simulink model "MSV_ablf"  (R2021a)
settings: Solver=ode4  StartTime=0.0  StopTime=10  FixedStep=0.001  MaxStep=0.01  RelTol=1e-3
model workspace (MAT data in the model file):
  EnableF = 1
  F_xyh = [10; 10; 1]
  GainKnownUncty = 1
  InputSat = [8591; 330.8; 839]
  InputSatOff = 1000
  Mmtx = [1  0  0; 0  1  0; 0  0  1]
  Temp = 0
  Test1 = Simulink.Parameter
  Test1.Value = 0
  Test1.DataType = 'auto'
  Test1.Dimensions = [1 1]
  boat_heading = 0
  boat_vel_x = 0
  boat_vel_y = 0
  earth_head = 2
  earth_x = 0
  earth_y = 2
  input_heading = 1
  input_x = 1
  input_y = 1
values from neighbouring files (symbols this model uses):
  Fval = [0 0 0]    [max_dist.m]    (also in test_ablf.m = [ ix iy iz ]; test_bs.m = [ ix iy iz ]; test_fxt.m = [ ix iy iz ]; test_max.m)
  LimStop = 0    [main.m]    (also in max_dist.m = 1)
libraries: dspmtrx3 x18, aerolibutil x4, simulink x1
(part 1 of 2)
settings Model: PacingRate=0.500000  ParameterArgumentNames=earth_head,earth_x,earth_y  OrderedModelArguments=off  Creator=14244039  LastModifiedBy=14244039
settings DebuggingCC: ReadBeforeWriteMsg=DisableAll
settings RTWCC: GenCodeOnly=on  BuildConfiguration=Faster Runs

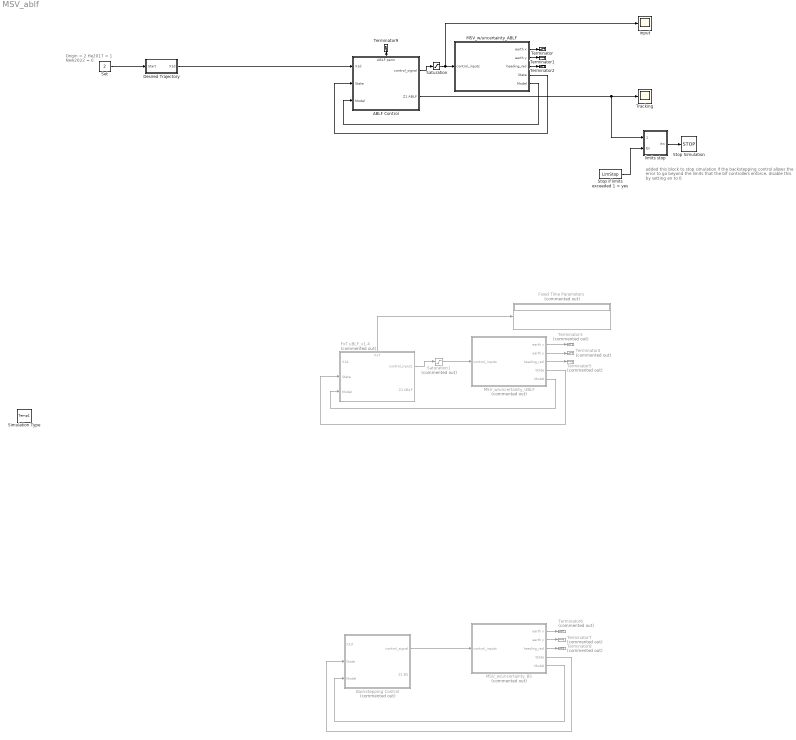
== system MSV_ablf ==
  note: Origin = 2
      | He2017 = 1
      | New2022 = 0
  note: added this block to stop simulation if the backstepping control allows
      | the error to go beyond the limits that the blf controllers enforce.
      | disable this by setting en to 0
  ABLF Control : Subsystem
      settings: PortSchema="{\"entries\":[{\"content\":{\"sides\":[{\"content\":{\"connectorIds\":[\"In1\",\"In2\",\"In3\"]},\"type\":\"ConnectorPlacement.EquallySpacedRectSide\",\"uuid\":\"f8e83fd1-45ec-473c-b127-dda3e39bc690\"},{\"content\":{\"connectorIds\":[\"Out1\",\"Out2\"],\"side\":\"RIGHT\"},\"type\":\"ConnectorPlacement.EquallySpacedRectSide\",\"uuid\":\"3907a693-0eb5-4391-af9e-fb1e42d629e6\"},{\"content\":{\"connectorIds\":[\"Out3\"],\"side\":\"TOP\"},\"type\":\"ConnectorPlacement.EquallySpacedRectSide\",\"uuid\":\"67f51e78-fb2e-4534-9eac-637fb7bc723a\"}]},\"type\":\"ConnectorPlacement.EquallySpacedConnector\",\"uuid\":\"eb746a93-d2ce-4178-8726-02b0a13fef5e\"}],\"packageUris\":[\"http://schema.mathworks.com/mf0/Connector/R2020b\"],\"version\":\"1.0\"}"
  Backstepping Control : Subsystem  Commented=on
  Desired Trajectory : Subsystem
  Fixed Time Parameters : Display  Commented=on
  FxT uBLF_v1.4 : Subsystem  Commented=on
      settings: PortSchema="{\"entries\":[{\"content\":{\"sides\":[{\"content\":{\"connectorIds\":[\"In1\",\"In2\",\"In3\"]},\"type\":\"ConnectorPlacement.EquallySpacedRectSide\",\"uuid\":\"f8e83fd1-45ec-473c-b127-dda3e39bc690\"},{\"content\":{\"connectorIds\":[\"Out1\",\"Out2\"],\"side\":\"RIGHT\"},\"type\":\"ConnectorPlacement.EquallySpacedRectSide\",\"uuid\":\"3907a693-0eb5-4391-af9e-fb1e42d629e6\"},{\"content\":{\"connectorIds\":[\"Out3\"],\"side\":\"TOP\"},\"type\":\"ConnectorPlacement.EquallySpacedRectSide\",\"uuid\":\"67f51e78-fb2e-4534-9eac-637fb7bc723a\"}]},\"type\":\"ConnectorPlacement.EquallySpacedConnector\",\"uuid\":\"eb746a93-d2ce-4178-8726-02b0a13fef5e\"}],\"packageUris\":[\"http://schema.mathworks.com/mf0/Connector/R2020b\"],\"version\":\"1.0\"}"
  MSV_w/uncertainty_ABLF : Subsystem
  MSV_w/uncertainty_BS : Subsystem  Commented=on
  MSV_w/uncertainty_UBLF : Subsystem  Commented=on
  Saturation : Saturate  UpperLimit=InputSat*InputSatOff  LowerLimit=-1*(InputSat)*InputSatOff
  Saturation1 : Saturate  Commented=on  UpperLimit=InputSat*InputSatOff  LowerLimit=-1*(InputSat)*InputSatOff
  Set : Constant  Value=2
  Simulation Type : DataStoreMemory  DataStoreName=Temp1  ReadBeforeWriteMsg=warning  WriteAfterWriteMsg=warning  WriteAfterReadMsg=warning  ShowAdditionalParam=off
  Stop Simulation : Stop
  Stop if limits exceeded 1 = yes : Constant  Value=LimStop
  Terminator{,1..2,9} (4 alike) : Terminator
  Terminator{3..8} (6 alike) : Terminator  Commented=on
  Tracking : Scope
  input : Scope
  limits stop : Subsystem
  wires:
  MSV_w/uncertainty_UBLF/4(State) -> FxT uBLF_v1.4/2(State)
  MSV_w/uncertainty_UBLF/5(Model) -> FxT uBLF_v1.4/3(Model)
  MSV_w/uncertainty_ABLF/4(State) -> ABLF Control/2(State)
  MSV_w/uncertainty_ABLF/5(Model) -> ABLF Control/3(Model)
  Set/1 -> Desired Trajectory/1(Start)
  FxT uBLF_v1.4/1(control_inputs) -> Saturation1/1
  ABLF Control/1(control_signal) -> Saturation/1
  Saturation1/1 -> MSV_w/uncertainty_UBLF/1(control_inputs)
  FxT uBLF_v1.4/3(FxT) -> Fixed Time Parameters/1
  Desired Trajectory/1(X1d) -> ABLF Control/1(X1d)
  Backstepping Control/1(control_signal) -> MSV_w/uncertainty_BS/1(control_inputs)
  MSV_w/uncertainty_BS/5(Model) -> Backstepping Control/3(Model)
  MSV_w/uncertainty_BS/4(State) -> Backstepping Control/2(State)
  MSV_w/uncertainty_ABLF/1(earth x) -> Terminator/1
  MSV_w/uncertainty_ABLF/2(earth y) -> Terminator1/1
  MSV_w/uncertainty_ABLF/3(heading_rad) -> Terminator2/1
  MSV_w/uncertainty_UBLF/1(earth x) -> Terminator3/1
  MSV_w/uncertainty_UBLF/2(earth y) -> Terminator4/1
  MSV_w/uncertainty_UBLF/3(heading_rad) -> Terminator5/1
  MSV_w/uncertainty_BS/1(earth x) -> Terminator6/1
  MSV_w/uncertainty_BS/2(earth y) -> Terminator7/1
  MSV_w/uncertainty_BS/3(heading_rad) -> Terminator8/1
  Saturation/1 -> input/1, MSV_w/uncertainty_ABLF/1(control_inputs)
  ABLF Control/3(ABLF parm) -> Terminator9/1
  limits stop/1(rtn) -> Stop Simulation/1
  ABLF Control/2(Z1 ABLF) -> limits stop/1(Z1 BS), Tracking/1
  Stop if limits exceeded 1 = yes/1 -> limits stop/2(En)

== system MSV_ablf/ABLF Control ==
  X1d : Inport
  State : Inport  Port=2
  Model : Inport  Port=3
  Constant : Constant  Value=0
  MATLAB Function : MATLAB Function  TreatAsAtomicUnit=on
  Selector : Selector  InputPortWidth=3  IndexOptions=Index vector (dialog)  Indices=1  OutputSizes=1
  Selector1 : Selector  InputPortWidth=3  IndexOptions=Index vector (dialog)  Indices=2  OutputSizes=1
  Selector2 : Selector  InputPortWidth=3  IndexOptions=Index vector (dialog)  Indices=3  OutputSizes=1
  State Feedback & Known Functions : Subsystem
  Terminator{,1..3} (4 alike) : Terminator
  u_ablf : Scope  NumInputPorts=3
  control_signal : Outport
  Z1 ABLF : Outport  Port=2
  ABLF parm : Outport  Port=3
  wires:
  State/1 -> State Feedback & Known Functions/2(State)
  State Feedback & Known Functions/1(C+D+G) -> MATLAB Function/1(CDG)
  State Feedback & Known Functions/2(M) -> MATLAB Function/2(M)
  State Feedback & Known Functions/5(X2) -> MATLAB Function/5(X2)
  State Feedback & Known Functions/4(X1) -> MATLAB Function/4(X1)
  State Feedback & Known Functions/3(J) -> MATLAB Function/3(J)
  Model/1 -> State Feedback & Known Functions/1(Model)
  X1d/1 -> MATLAB Function/6(X1d)  "xd"
  MATLAB Function/6(test2) -> Z1 ABLF/1
  MATLAB Function/7(pABLF) -> ABLF parm/1
  Selector/1 -> u_ablf/1  "uLong"
  MATLAB Function/1(u) -> control_signal/1, Selector/1, Selector1/1, Selector2/1
  Selector1/1 -> u_ablf/2  "uLateral"
  Selector2/1 -> u_ablf/3  "uRotate"
  Constant/1 -> MATLAB Function/8(unused1), MATLAB Function/7(unused)
  MATLAB Function/2(x_Err) -> Terminator/1
  MATLAB Function/3(y_Err) -> Terminator1/1
  MATLAB Function/4(h_Err) -> Terminator2/1
  MATLAB Function/5(test1) -> Terminator3/1

== system MSV_ablf/Backstepping Control ==
  X1d : Inport
  State : Inport  Port=2
  Model : Inport  Port=3
  Constant : Constant
  MATLAB Function : MATLAB Function  TreatAsAtomicUnit=on
  Selector : Selector  InputPortWidth=3  IndexOptions=Index vector (dialog)  Indices=1  OutputSizes=1
  Selector1 : Selector  InputPortWidth=3  IndexOptions=Index vector (dialog)  Indices=2  OutputSizes=1
  Selector2 : Selector  InputPortWidth=3  IndexOptions=Index vector (dialog)  Indices=3  OutputSizes=1
  State Feedback & Known Functions : Subsystem
  Terminator{,1..3} (4 alike) : Terminator
  u_bs : Scope  NumInputPorts=3
  control_signal : Outport
  Z1 BS : Outport  Port=2
  wires:
  State/1 -> State Feedback & Known Functions/2(State)
  State Feedback & Known Functions/1(C+D+G) -> MATLAB Function/1(CDG)
  State Feedback & Known Functions/2(M) -> MATLAB Function/2(M)
  State Feedback & Known Functions/5(X2) -> MATLAB Function/5(X2)
  State Feedback & Known Functions/4(X1) -> MATLAB Function/4(X1)
  State Feedback & Known Functions/3(J) -> MATLAB Function/3(J)
  Model/1 -> State Feedback & Known Functions/1(Model)
  X1d/1 -> MATLAB Function/6(X1d)  "xd"
  MATLAB Function/6(test2) -> Z1 BS/1
  Selector/1 -> u_bs/1  "uLong"
  MATLAB Function/1(u) -> Selector/1, Selector1/1, Selector2/1, control_signal/1
  Selector1/1 -> u_bs/2  "uLateral"
  Selector2/1 -> u_bs/3  "uRotate"
  Constant/1 -> MATLAB Function/8(unused1), MATLAB Function/7(unused)
  MATLAB Function/2(x_Err) -> Terminator/1
  MATLAB Function/3(y_Err) -> Terminator1/1
  MATLAB Function/4(h_Err) -> Terminator2/1
  MATLAB Function/5(test1) -> Terminator3/1

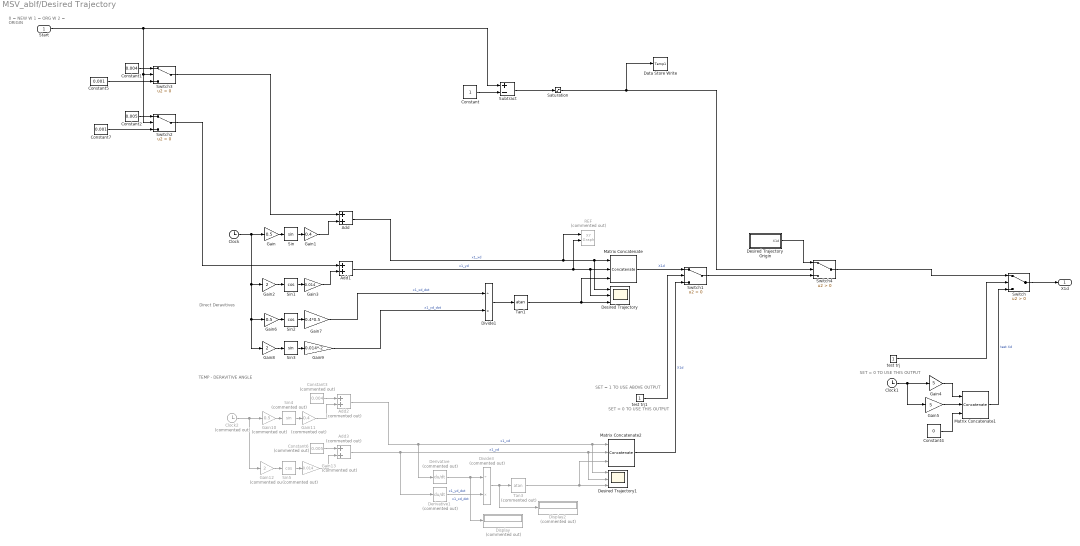
== system MSV_ablf/Desired Trajectory ==
  note: 0 = NEW W
      | 1 = ORG W
      | 2 = ORIGIN
  note: Direct Deravitives
  note: SET = 0 TO USE THIS OUTPUT
  note: TEMP - DERAVITIVE ANGLE
  note: SET = 1 TO USE ABOVE OUTPUT
  note: SET = 0 TO USE THIS OUTPUT
  Start : Inport
  Add : Sum
  Add1 : Sum
  Add2 : Sum  Commented=on
  Add3 : Sum  Commented=on
  Clock : Clock
  Clock1 : Clock
  Clock2 : Clock  Commented=on
  Constant : Constant
  Constant1 : Constant  Value=0.004
  Constant2 : Constant  Value=0.005
  Constant3 : Constant  Commented=on  Value=0.004
  Constant4 : Constant  Value=0
  Constant5 : Constant  Value=0.001
  Constant6 : Constant  Commented=on  Value=0.005
  Constant7 : Constant  Value=0.001
  Data Store Write : DataStoreWrite  DataStoreName=Temp1  IndexOptions=Index vector (dialog)  Indices=1  OutputSizes=1
  Derivative : Derivative  Commented=on
  Derivative1 : Derivative  Commented=on
  Desired Trajectory : Scope  NumInputPorts=3
  Desired Trajectory Origin : Subsystem
  Desired Trajectory1 : Scope  NumInputPorts=3
  Display : Display  Commented=on
  Display2 : Display  Commented=on
  Divide1 : Product  Inputs=/*
  Divide3 : Product  Commented=on  Inputs=/*
  Gain : Gain  Gain=0.5
  Gain1 : Gain  Gain=0.4
  Gain10 : Gain  Commented=on  Gain=0.5
  Gain11 : Gain  Commented=on  Gain=0.4
  Gain12 : Gain  Commented=on  Gain=2
  Gain13 : Gain  Commented=on  Gain=0.014
  Gain2 : Gain  Gain=2
  Gain3 : Gain  Gain=0.014
  Gain4 : Gain  Gain=5
  Gain5 : Gain  Gain=5
  Gain6 : Gain  Gain=0.5
  Gain7 : Gain  Gain=0.4*0.5
  Gain8 : Gain  Gain=2
  Gain9 : Gain  Gain=0.014*-2
  Matrix Concatenate : Concatenate  NumInputs=3  Mode=Multidimensional array
  Matrix Concatenate1 : Concatenate  NumInputs=3  Mode=Multidimensional array
  Matrix Concatenate2 : Concatenate  NumInputs=3  Mode=Multidimensional array
  REF : simulink/Sinks/XY Graph  Commented=on  xmin=-0.65  xmax=0.65  ymin=-0.012  ymax=0.022  st=-1
  Saturation : Saturate  UpperLimit=1
  Sin : Trigonometry
  Sin1 : Trigonometry  Operator=cos
  Sin2 : Trigonometry  Operator=cos
  Sin3 : Trigonometry
  Sin4 : Trigonometry  Commented=on
  Sin5 : Trigonometry  Commented=on  Operator=cos
  Subtract : Sum  Inputs=+-
  Switch{,1..4} (5 alike) : Switch  Criteria=u2 > Threshold
  Tan1 : Trigonometry  Operator=atan  ApproximationMethod=CORDIC  OutputSignalType=real
  Tan3 : Trigonometry  Commented=on  Operator=atan  ApproximationMethod=CORDIC  OutputSignalType=real
  test trj : Constant
  test trj1 : Constant
  X1d : Outport
  wires:
  Clock/1 -> Gain/1, Gain8/1, Gain6/1, Gain2/1
  Switch3/1 -> Add/1
  Sin/1 -> Gain1/1
  Gain/1 -> Sin/1
  Add1/1 -> Matrix Concatenate/2, Desired Trajectory/2, REF/2  "x1_yd"
  Gain1/1 -> Add/2
  Switch2/1 -> Add1/1
  Gain2/1 -> Sin1/1
  Add/1 -> REF/1, Desired Trajectory/1, Matrix Concatenate/1  "x1_xd"
  Gain3/1 -> Add1/2
  Sin1/1 -> Gain3/1
  Matrix Concatenate/1 -> Switch1/1  "X1d"
  Gain9/1 -> Divide1/2  "x1_yd_dot"
  Tan1/1 -> Matrix Concatenate/3, Desired Trajectory/3
  Switch/1 -> X1d/1
  test trj/1 -> Switch/2
  Matrix Concatenate1/1 -> Switch/3  "test Xd"
  Gain5/1 -> Matrix Concatenate1/2
  Gain4/1 -> Matrix Concatenate1/1
  Clock1/1 -> Gain5/1, Gain4/1
  Constant4/1 -> Matrix Concatenate1/3
  Gain7/1 -> Divide1/1  "x1_xd_dot"
  Divide1/1 -> Tan1/1
  Gain6/1 -> Sin2/1
  Sin2/1 -> Gain7/1
  Sin3/1 -> Gain9/1
  Gain8/1 -> Sin3/1
  Divide3/1 -> Display2/1, Tan3/1
  Derivative/1 -> Display/1, Divide3/1  "x1_xd_dot"
  Tan3/1 -> Desired Trajectory1/3, Matrix Concatenate2/3
  Derivative1/1 -> Divide3/2  "x1_yd_dot"
  Sin5/1 -> Gain13/1
  Gain13/1 -> Add3/2
  Add2/1 -> Derivative/1, Matrix Concatenate2/1, Desired Trajectory1/1  "x1_xd"
  Gain12/1 -> Sin5/1
  Constant6/1 -> Add3/1
  Gain11/1 -> Add2/2
  Add3/1 -> Derivative1/1, Matrix Concatenate2/2, Desired Trajectory1/2  "x1_yd"
  Gain10/1 -> Sin4/1
  Sin4/1 -> Gain11/1
  Constant3/1 -> Add2/1
  Clock2/1 -> Gain12/1, Gain10/1
  Switch4/1 -> Switch/1
  Matrix Concatenate2/1 -> Switch1/3  "X1d"
  test trj1/1 -> Switch1/2
  Constant2/1 -> Switch2/1
  Constant1/1 -> Switch3/1
  Constant5/1 -> Switch3/3
  Constant7/1 -> Switch2/3
  Switch1/1 -> Switch4/3
  Desired Trajectory Origin/1(X1d) -> Switch4/1
  Subtract/1 -> Saturation/1
  Constant/1 -> Subtract/2
  Start/1 -> Switch2/2, Switch3/2, Subtract/1
  Saturation/1 -> Data Store Write/1, Switch4/2

== system MSV_ablf/FxT uBLF_v1.4 ==
  X1d : Inport
  State : Inport  Port=2
  Model : Inport  Port=3
  Constant : Constant  Value=0
  Control Signals : Scope  NumInputPorts=3
  Fixed Time Tmax : Display
  Selector : Selector  InputPortWidth=3  IndexOptions=Index vector (dialog)  Indices=1  OutputSizes=1
  Selector1 : Selector  InputPortWidth=3  IndexOptions=Index vector (dialog)  Indices=2  OutputSizes=1
  Selector2 : Selector  InputPortWidth=3  IndexOptions=Index vector (dialog)  Indices=3  OutputSizes=1
  Selector3 : Selector  InputPortWidth=9  IndexOptions=Index vector (dialog)  Indices=1  OutputSizes=1
  State Feedback & Known Functions : Subsystem
  SymUBLF1 : MATLAB Function  Commented=on  TreatAsAtomicUnit=on
  Terminator : Terminator
  Terminator1 : Terminator
  Terminator2 : Terminator
  UBLF : MATLAB Function  TreatAsAtomicUnit=on
  control_inputs : Outport
  Z1 UBLF : Outport  Port=2
  FxT : Outport  Port=3
  wires:
  X1d/1 -> UBLF/6(Xd)  "X1d"
  Model/1 -> State Feedback & Known Functions/1(Model)
  State/1 -> State Feedback & Known Functions/2(State)
  State Feedback & Known Functions/1(F2) -> UBLF/1(F2)
  State Feedback & Known Functions/2(G2) -> UBLF/2(G2)
  State Feedback & Known Functions/3(G1) -> UBLF/3(G1)
  State Feedback & Known Functions/4(X1) -> UBLF/4(X1)
  State Feedback & Known Functions/5(X2) -> UBLF/5(X2)
  Selector/1 -> Control Signals/1  "uLong"
  Selector1/1 -> Control Signals/2  "uLateral"
  Selector2/1 -> Control Signals/3  "uRotate"
  UBLF/1(u) -> control_inputs/1, Selector1/1, Selector2/1, Selector/1
  UBLF/5(test1) -> Z1 UBLF/1
  UBLF/6(test2) -> FxT/1, Selector3/1
  Selector3/1 -> Fixed Time Tmax/1
  Constant/1 -> UBLF/8(unused1), UBLF/7(unused)
  UBLF/2(xErr) -> Terminator/1
  UBLF/3(yErr) -> Terminator1/1
  UBLF/4(hErr) -> Terminator2/1

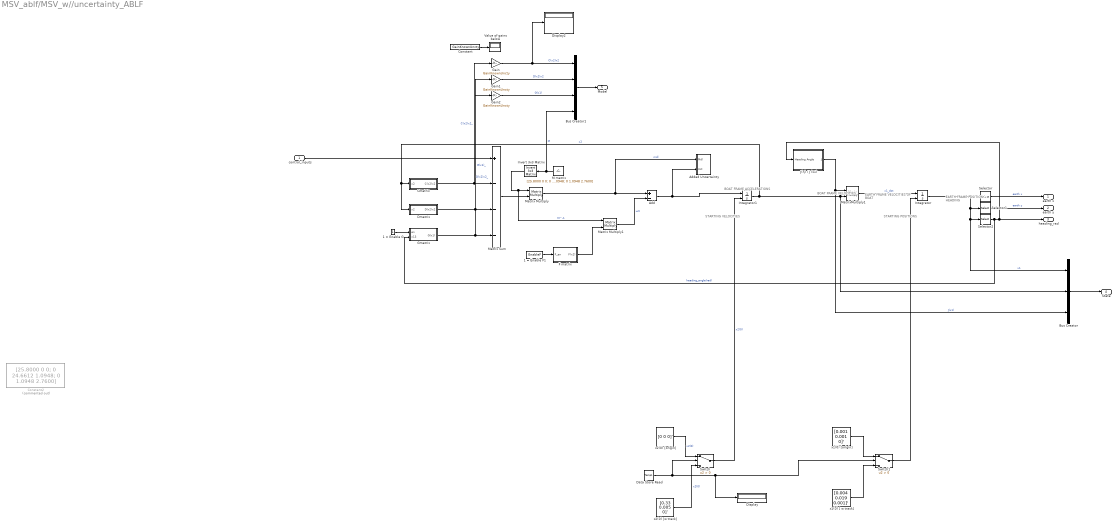
== system MSV_ablf/MSV_w//uncertainty_ABLF ==
  note: STARTING VELOCITIES
  note: STARTING POSITIONS
  note: BOAT FRAME
      | ACCELERATIONS
  note: BOAT FRAME
      | VELOCITIES
  note: EARTH FRAME
      | VELOCITIES OF BOAT
  note: EARTH FRAME
      | POSITION + HEADING
  control_inputs : Inport
  1 = Enable F1 : Constant  Value=EnableF
  1 = Enable G : Constant
  Add : Sum  Inputs=+-
  Added Uncertainty : Subsystem
  Bus Creator : BusCreator  Inputs=3
  Bus Creator1 : BusCreator  Inputs=4
  Cmatrix : Subsystem
  Constant : Constant  Value=GainKnownUncty
  Constant2 : Constant  Commented=on  Value=[25.8000 0 0; 0 24.6612 1.0948; 0 1.0948 2.7600]  VectorParams1D=off
  Data Store Read : DataStoreRead  DataStoreName=Temp1  IndexOptions=Index vector (dialog)  Indices=1  OutputSizes=1
  Display : Display
  Display2 : Display
  Dmatrix : Subsystem
  F matrix : Subsystem
  Gain : Gain  Gain=GainKnownUncty
  Gain1 : Gain  Gain=GainKnownUncty
  Gain2 : Gain  Gain=GainKnownUncty
  Gmatrix : Subsystem
  Integrator : Integrator  InitialConditionSource=external
  Integrator1 : Integrator  InitialConditionSource=external  IgnoreLimit=on
  Invert 3x3 Matrix : aerolibutil/Invert  3x3 Matrix
  J(η) / J (x1) : Subsystem
  M matrix : Constant  Value=[25.8000 0 0; 0 24.6612 1.0948; 0 1.0948 2.7600]  VectorParams1D=off
  Matrix Sum : Sum  Inputs=+---
  Matrix Multiply : Product  Multiplication=Matrix(*)
  Matrix Multiply1 : Product  Multiplication=Matrix(*)
  MatrixMultiply1 : Product  Multiplication=Matrix(*)
  Selector : Selector  InputPortWidth=3  IndexOptions=Index vector (dialog)  Indices=1  OutputSizes=1
  Selector1 : Selector  InputPortWidth=3  IndexOptions=Index vector (dialog)  Indices=2  OutputSizes=1
  Selector2 : Selector  InputPortWidth=3  IndexOptions=Index vector (dialog)  Indices=3  OutputSizes=1
  Switch : Switch  Criteria=u2 > Threshold
  Switch1 : Switch  Criteria=u2 > Threshold
  Value of gains below : Display
  x1(0) [ w track] : Constant  Value=[0.004 0.019 0.001]'  VectorParams1D=off
  x1(0) [origin] : Constant  Value=[0.001 0.001 0]'  VectorParams1D=off
  x2(0) [origin] : Constant  Value=[0 0 0]'  VectorParams1D=off
  x2(0) [w track] : Constant  Value=[0.33 0.005 0]'  VectorParams1D=off
  earth x : Outport
  earth y : Outport  Port=2
  heading_rad : Outport  Port=3
  State : Outport  Port=4
  Model : Outport  Port=5
  wires:
  Gain2/1 -> Bus Creator1/3  "G(x1)"
  Gain1/1 -> Bus Creator1/2  "D(x2)x2"
  Gain/1 -> Bus Creator1/1, Display2/1  "C(x2)x2"
  F matrix/1(F(x2)) -> Matrix Multiply1/2
  1 = Enable F1/1 -> F matrix/1(F_en)
  Add/1 -> Integrator1/1, Added Uncertainty/2(Uct)
  Matrix Multiply1/1 -> Add/2  "uct"
  Bus Creator1/1 -> Model/1
  Bus Creator/1 -> State/1
  Cmatrix/1(C(x2)x2) -> Matrix Sum/2, Gain/1  "C(x2)x2_"
  Switch/1 -> Integrator1/2  "x2(0)"
  Integrator1/1 -> Cmatrix/1(x2), Dmatrix/1(x2), MatrixMultiply1/2, Bus Creator/2  "x2"
  1 = Enable G/1 -> Gmatrix/1(en)
  Selector2/1 -> Gmatrix/2(x13), J(η) / J (x1)/1(Heading Angle), heading_rad/1  "heading_angle(rad)"
  Selector/1 -> earth x/1  "earth x"
  Selector1/1 -> earth y/1  "earth y"
  Gmatrix/1(G(x1)) -> Gain2/1, Matrix Sum/4  "G(x1)_"
  Invert 3x3 Matrix/1 -> Matrix Multiply/1, Matrix Multiply1/1  "M^-1"
  Dmatrix/1(D(x2)x2) -> Matrix Sum/3, Gain1/1  "D(x2)x2_"
  Integrator/1 -> Selector/1, Selector1/1, Selector2/1, Bus Creator/1  "x1"
  MatrixMultiply1/1 -> Integrator/1  "x1_dot"
  M matrix/1 -> Invert 3x3 Matrix/1, Bus Creator1/4  "M"
  J(η) / J (x1)/1(J) -> MatrixMultiply1/1, Bus Creator/3  "J(x1)"
  Matrix Multiply/1 -> Add/1, Added Uncertainty/1(Mdl)  "mdl"
  Matrix Sum/1 -> Matrix Multiply/2
  Constant/1 -> Value of gains below/1
  control_inputs/1 -> Matrix Sum/1
  Switch1/1 -> Integrator/2
  x2(0) [origin]/1 -> Switch/1  "x2(0)"
  x2(0) [w track]/1 -> Switch/3  "x2(0)"
  x1(0) [origin]/1 -> Switch1/1
  x1(0) [ w track]/1 -> Switch1/3
  Data Store Read/1 -> Switch/2, Display/1, Switch1/2

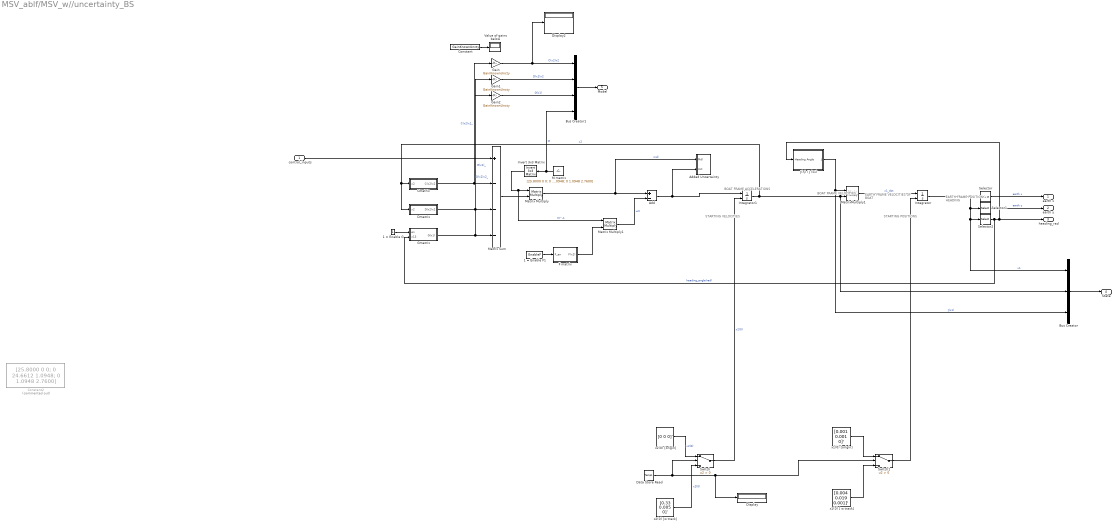
== system MSV_ablf/MSV_w//uncertainty_BS ==
  note: EARTH FRAME
      | POSITION + HEADING
  note: EARTH FRAME
      | VELOCITIES OF BOAT
  note: BOAT FRAME
      | VELOCITIES
  note: BOAT FRAME
      | ACCELERATIONS
  note: STARTING POSITIONS
  note: STARTING VELOCITIES
  control_inputs : Inport
  1 = Enable F1 : Constant  Value=EnableF
  1 = Enable G : Constant
  Add : Sum  Inputs=+-
  Added Uncertainty : Subsystem
  Bus Creator : BusCreator  Inputs=3
  Bus Creator1 : BusCreator  Inputs=4
  Cmatrix : Subsystem
  Constant : Constant  Value=GainKnownUncty
  Constant2 : Constant  Commented=on  Value=[25.8000 0 0; 0 24.6612 1.0948; 0 1.0948 2.7600]  VectorParams1D=off
  Data Store Read : DataStoreRead  DataStoreName=Temp1  IndexOptions=Index vector (dialog)  Indices=1  OutputSizes=1
  Display : Display
  Display2 : Display
  Dmatrix : Subsystem
  F matrix : Subsystem
  Gain : Gain  Gain=GainKnownUncty
  Gain1 : Gain  Gain=GainKnownUncty
  Gain2 : Gain  Gain=GainKnownUncty
  Gmatrix : Subsystem
  Integrator : Integrator  InitialConditionSource=external
  Integrator1 : Integrator  InitialConditionSource=external  IgnoreLimit=on
  Invert 3x3 Matrix : aerolibutil/Invert  3x3 Matrix
  J(η) / J (x1) : Subsystem
  M matrix : Constant  Value=[25.8000 0 0; 0 24.6612 1.0948; 0 1.0948 2.7600]  VectorParams1D=off
  Matrix Sum : Sum  Inputs=+---
  Matrix Multiply : Product  Multiplication=Matrix(*)
  Matrix Multiply1 : Product  Multiplication=Matrix(*)
  MatrixMultiply1 : Product  Multiplication=Matrix(*)
  Selector : Selector  InputPortWidth=3  IndexOptions=Index vector (dialog)  Indices=1  OutputSizes=1
  Selector1 : Selector  InputPortWidth=3  IndexOptions=Index vector (dialog)  Indices=2  OutputSizes=1
  Selector2 : Selector  InputPortWidth=3  IndexOptions=Index vector (dialog)  Indices=3  OutputSizes=1
  Switch : Switch  Criteria=u2 > Threshold
  Switch1 : Switch  Criteria=u2 > Threshold
  Value of gains below : Display
  x1(0) [ w track] : Constant  Value=[0.004 0.019 0.001]'  VectorParams1D=off
  x1(0) [origin] : Constant  Value=[0.001 0.001 0]'  VectorParams1D=off
  x2(0) [origin] : Constant  Value=[0 0 0]'  VectorParams1D=off
  x2(0) [w track] : Constant  Value=[0.33 0.005 0]'  VectorParams1D=off
  earth x : Outport
  earth y : Outport  Port=2
  heading_rad : Outport  Port=3
  State : Outport  Port=4
  Model : Outport  Port=5
  wires:
  Data Store Read/1 -> Switch1/2, Display/1, Switch/2
  x1(0) [ w track]/1 -> Switch1/3
  x1(0) [origin]/1 -> Switch1/1
  x2(0) [w track]/1 -> Switch/3  "x2(0)"
  x2(0) [origin]/1 -> Switch/1  "x2(0)"
  Switch1/1 -> Integrator/2
  control_inputs/1 -> Matrix Sum/1
  Constant/1 -> Value of gains below/1
  Matrix Sum/1 -> Matrix Multiply/2
  Matrix Multiply/1 -> Added Uncertainty/1(Mdl), Add/1  "mdl"
  J(η) / J (x1)/1(J) -> Bus Creator/3, MatrixMultiply1/1  "J(x1)"
  M matrix/1 -> Bus Creator1/4, Invert 3x3 Matrix/1  "M"
  MatrixMultiply1/1 -> Integrator/1  "x1_dot"
  Integrator/1 -> Bus Creator/1, Selector2/1, Selector1/1, Selector/1  "x1"
  Dmatrix/1(D(x2)x2) -> Gain1/1, Matrix Sum/3  "D(x2)x2_"
  Invert 3x3 Matrix/1 -> Matrix Multiply1/1, Matrix Multiply/1  "M^-1"
  Gmatrix/1(G(x1)) -> Matrix Sum/4, Gain2/1  "G(x1)_"
  Selector1/1 -> earth y/1  "earth y"
  Selector/1 -> earth x/1  "earth x"
  Selector2/1 -> heading_rad/1, J(η) / J (x1)/1(Heading Angle), Gmatrix/2(x13)  "heading_angle(rad)"
  1 = Enable G/1 -> Gmatrix/1(en)
  Integrator1/1 -> Bus Creator/2, MatrixMultiply1/2, Dmatrix/1(x2), Cmatrix/1(x2)  "x2"
  Switch/1 -> Integrator1/2  "x2(0)"
  Cmatrix/1(C(x2)x2) -> Gain/1, Matrix Sum/2  "C(x2)x2_"
  Bus Creator/1 -> State/1
  Bus Creator1/1 -> Model/1
  Matrix Multiply1/1 -> Add/2  "uct"
  Add/1 -> Added Uncertainty/2(Uct), Integrator1/1
  1 = Enable F1/1 -> F matrix/1(F_en)
  F matrix/1(F(x2)) -> Matrix Multiply1/2
  Gain/1 -> Display2/1, Bus Creator1/1  "C(x2)x2"
  Gain1/1 -> Bus Creator1/2  "D(x2)x2"
  Gain2/1 -> Bus Creator1/3  "G(x1)"

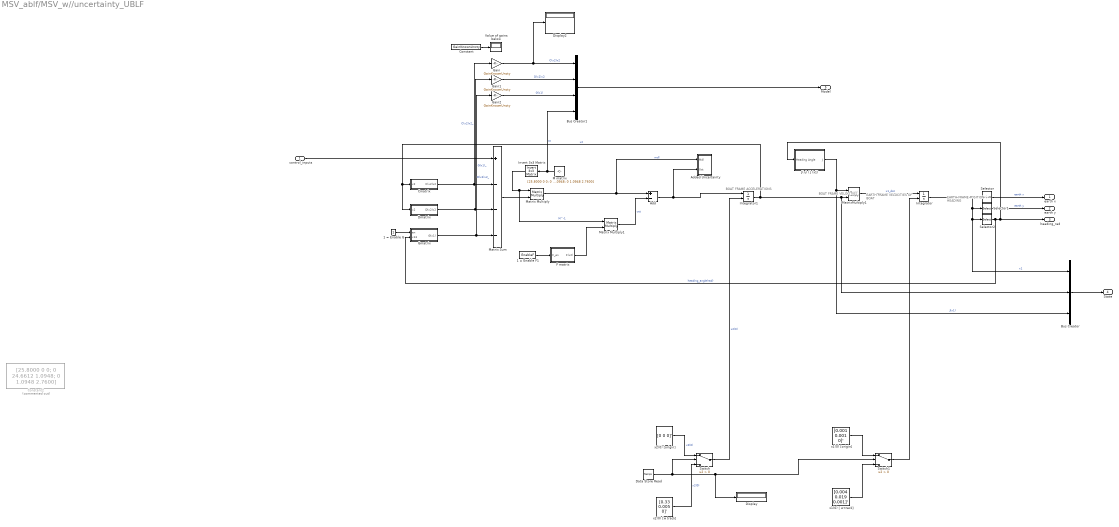
== system MSV_ablf/MSV_w//uncertainty_UBLF ==
  note: EARTH FRAME
      | POSITION + HEADING
  note: EARTH FRAME
      | VELOCITIES OF BOAT
  note: BOAT FRAME
      | VELOCITIES
  note: BOAT FRAME
      | ACCELERATIONS
  control_inputs : Inport
  1 = Enable F1 : Constant  Value=EnableF
  1 = Enable G : Constant
  Add : Sum  Inputs=+-
  Added Uncertainty : Subsystem
  Bus Creator : BusCreator  Inputs=3
  Bus Creator1 : BusCreator  Inputs=4
  Cmatrix : Subsystem
  Constant : Constant  Value=GainKnownUncty
  Constant2 : Constant  Commented=on  Value=[25.8000 0 0; 0 24.6612 1.0948; 0 1.0948 2.7600]  VectorParams1D=off
  Data Store Read : DataStoreRead  DataStoreName=Temp1  IndexOptions=Index vector (dialog)  Indices=1  OutputSizes=1
  Display : Display
  Display2 : Display
  Dmatrix : Subsystem
  F matrix : Subsystem
  Gain : Gain  Gain=GainKnownUncty
  Gain1 : Gain  Gain=GainKnownUncty
  Gain2 : Gain  Gain=GainKnownUncty
  Gmatrix : Subsystem
  Integrator : Integrator  InitialConditionSource=external
  Integrator1 : Integrator  InitialConditionSource=external  IgnoreLimit=on
  Invert 3x3 Matrix : aerolibutil/Invert  3x3 Matrix
  J(η) / J (x1) : Subsystem
  M matrix : Constant  Value=[25.8000 0 0; 0 24.6612 1.0948; 0 1.0948 2.7600]  VectorParams1D=off
  Matrix Sum : Sum  Inputs=+---
  Matrix Multiply : Product  Multiplication=Matrix(*)
  Matrix Multiply1 : Product  Multiplication=Matrix(*)
  MatrixMultiply1 : Product  Multiplication=Matrix(*)
  Selector : Selector  InputPortWidth=3  IndexOptions=Index vector (dialog)  Indices=1  OutputSizes=1
  Selector1 : Selector  InputPortWidth=3  IndexOptions=Index vector (dialog)  Indices=2  OutputSizes=1
  Selector2 : Selector  InputPortWidth=3  IndexOptions=Index vector (dialog)  Indices=3  OutputSizes=1
  Switch : Switch  Criteria=u2 > Threshold
  Switch1 : Switch  Criteria=u2 > Threshold
  Value of gains below : Display
  x1(0) [ w track] : Constant  Value=[0.004 0.019 0.001]'  VectorParams1D=off
  x1(0) [origin] : Constant  Value=[0.001 0.001 0]'  VectorParams1D=off
  x2(0) [origin] : Constant  Value=[0 0 0]'  VectorParams1D=off
  x2(0) [w track] : Constant  Value=[0.33 0.005 0]'  VectorParams1D=off
  earth x : Outport
  earth y : Outport  Port=2
  heading_rad : Outport  Port=3
  State : Outport  Port=4
  Model : Outport  Port=5
  wires:
  control_inputs/1 -> Matrix Sum/1
  Constant/1 -> Value of gains below/1
  Matrix Sum/1 -> Matrix Multiply/2
  Matrix Multiply/1 -> Added Uncertainty/1(Mdl), Add/1  "mdl"
  J(η) / J (x1)/1(J) -> Bus Creator/3, MatrixMultiply1/1  "J(x1)"
  M matrix/1 -> Bus Creator1/4, Invert 3x3 Matrix/1  "M"
  MatrixMultiply1/1 -> Integrator/1  "x1_dot"
  Integrator/1 -> Bus Creator/1, Selector2/1, Selector1/1, Selector/1  "x1"
  Dmatrix/1(D(x2)x2) -> Gain1/1, Matrix Sum/3  "D(x2)x2_"
  Invert 3x3 Matrix/1 -> Matrix Multiply1/1, Matrix Multiply/1  "M^-1"
  Gmatrix/1(G(x1)) -> Matrix Sum/4, Gain2/1  "G(x1)_"
  Selector1/1 -> earth y/1  "earth y"
  Selector/1 -> earth x/1  "earth x"
  Selector2/1 -> heading_rad/1, J(η) / J (x1)/1(Heading Angle), Gmatrix/2(x13)  "heading_angle(rad)"
  1 = Enable G/1 -> Gmatrix/1(en)
  Integrator1/1 -> Bus Creator/2, MatrixMultiply1/2, Dmatrix/1(x2), Cmatrix/1(x2)  "x2"
  Cmatrix/1(C(x2)x2) -> Gain/1, Matrix Sum/2  "C(x2)x2_"
  Bus Creator/1 -> State/1
  Bus Creator1/1 -> Model/1
  Matrix Multiply1/1 -> Add/2  "uct"
  Add/1 -> Added Uncertainty/2(Uct), Integrator1/1
  1 = Enable F1/1 -> F matrix/1(F_en)
  F matrix/1(F(x2)) -> Matrix Multiply1/2
  Gain/1 -> Display2/1, Bus Creator1/1  "C(x2)x2"
  Gain1/1 -> Bus Creator1/2  "D(x2)x2"
  Gain2/1 -> Bus Creator1/3  "G(x1)"
  x1(0) [origin]/1 -> Switch1/1
  x2(0) [w track]/1 -> Switch/3  "x2(0)"
  Switch1/1 -> Integrator/2
  x2(0) [origin]/1 -> Switch/1  "x2(0)"
  Switch/1 -> Integrator1/2  "x2(0)"
  Data Store Read/1 -> Switch/2, Display/1, Switch1/2
  x1(0) [ w track]/1 -> Switch1/3

== system MSV_ablf/limits stop ==
  Z1 BS : Inport
  En : Inport  Port=2
  MATLAB Function : MATLAB Function  TreatAsAtomicUnit=on
  rtn : Outport
  wires:
  Z1 BS/1 -> MATLAB Function/1(Z1)
  En/1 -> MATLAB Function/2(en)
  MATLAB Function/1(rtn) -> rtn/1

== system MSV_ablf/ABLF Control/State Feedback & Known Functions ==
  Model : Inport
  State : Inport  Port=2
  Add : Sum  Inputs=+++
  Bus Selector : BusSelector  OutputSignals=C(x2)x2,D(x2)x2,G(x1),M
  Bus Selector1 : BusSelector  OutputSignals=J(x1),x1,x2
  Display : Display
  C+D+G : Outport
  M : Outport  Port=2
  J : Outport  Port=3
  X1 : Outport  Port=4
  X2 : Outport  Port=5
  wires:
  Bus Selector/2 -> Add/2  "<D(x2)x2>"
  Bus Selector/3 -> Add/3  "<G(x1)>"
  Bus Selector/1 -> Add/1  "<C(x2)x2>"
  State/1 -> Bus Selector1/1
  Bus Selector/4 -> M/1  "<M>"
  Bus Selector1/1 -> J/1  "<J(x1)>"
  Model/1 -> Bus Selector/1
  Bus Selector1/2 -> X1/1  "<x1>"
  Bus Selector1/3 -> X2/1  "<x2>"
  Add/1 -> Display/1, C+D+G/1

== system MSV_ablf/Backstepping Control/State Feedback & Known Functions ==
  Model : Inport
  State : Inport  Port=2
  Add : Sum  Inputs=---
  Bus Selector : BusSelector  OutputSignals=C(x2)x2,D(x2)x2,G(x1),M
  Bus Selector1 : BusSelector  OutputSignals=J(x1),x1,x2
  Display : Display
  C+D+G : Outport
  M : Outport  Port=2
  J : Outport  Port=3
  X1 : Outport  Port=4
  X2 : Outport  Port=5
  wires:
  Bus Selector/2 -> Add/2  "<D(x2)x2>"
  Bus Selector/3 -> Add/3  "<G(x1)>"
  Bus Selector/1 -> Add/1  "<C(x2)x2>"
  State/1 -> Bus Selector1/1
  Bus Selector/4 -> M/1  "<M>"
  Bus Selector1/1 -> J/1  "<J(x1)>"
  Model/1 -> Bus Selector/1
  Bus Selector1/2 -> X1/1  "<x1>"
  Bus Selector1/3 -> X2/1  "<x2>"
  Add/1 -> Display/1, C+D+G/1

== system MSV_ablf/Desired Trajectory/Desired Trajectory Origin ==
  Constant : Constant  Value=[0.0012 0.0012 0]'  VectorParams1D=off
  X1d : Outport
  wires:
  Constant/1 -> X1d/1  "X1d"

== system MSV_ablf/FxT uBLF_v1.4/State Feedback & Known Functions ==
  Model : Inport
  State : Inport  Port=2
  Add : Sum  Inputs=---
  Bus Selector : BusSelector  OutputSignals=C(x2)x2,D(x2)x2,G(x1),M
  Bus Selector1 : BusSelector  OutputSignals=J(x1),x1,x2
  Gain : Gain
  Gain1 : Gain
  Invert 3x3 Matrix : aerolibutil/Invert  3x3 Matrix
  Matrix Multiply : Product  Multiplication=Matrix(*)
  F2 : Outport
  G2 : Outport  Port=2
  G1 : Outport  Port=3
  X1 : Outport  Port=4
  X2 : Outport  Port=5
  wires:
  Bus Selector/2 -> Add/2  "<D(x2)x2>"
  Invert 3x3 Matrix/1 -> Gain/1, Matrix Multiply/1  "M^-1"
  Bus Selector/3 -> Add/3  "<G(x1)>"
  Matrix Multiply/1 -> F2/1  "f2"
  Bus Selector/1 -> Add/1  "<C(x2)x2>"
  State/1 -> Bus Selector1/1
  Add/1 -> Matrix Multiply/2
  Bus Selector/4 -> Invert 3x3 Matrix/1  "<M>"
  Bus Selector1/1 -> Gain1/1  "<J(x1)>"
  Model/1 -> Bus Selector/1
  Gain/1 -> G2/1  "g2"
  Gain1/1 -> G1/1  "g1"
  Bus Selector1/2 -> X1/1  "<x1>"
  Bus Selector1/3 -> X2/1  "<x2>"

== system MSV_ablf/MSV_w//uncertainty_ABLF/Added Uncertainty ==
  Mdl : Inport
  Uct : Inport  Port=2
  Scope : Scope  NumInputPorts=3
  Selector : Selector  InputPortWidth=3  IndexOptions=Index vector (dialog)  Indices=1  OutputSizes=1
  Selector1 : Selector  InputPortWidth=3  IndexOptions=Index vector (dialog)  Indices=1  OutputSizes=1
  Selector2 : Selector  InputPortWidth=3  IndexOptions=Index vector (dialog)  Indices=2  OutputSizes=1
  Selector3 : Selector  InputPortWidth=3  IndexOptions=Index vector (dialog)  Indices=2  OutputSizes=1
  Selector4 : Selector  InputPortWidth=3  IndexOptions=Index vector (dialog)  Indices=3  OutputSizes=1
  Selector5 : Selector  InputPortWidth=3  IndexOptions=Index vector (dialog)  Indices=3  OutputSizes=1
  Vector Concatenate : Concatenate
  Vector Concatenate1 : Concatenate
  Vector Concatenate2 : Concatenate
  wires:
  Mdl/1 -> Selector/1, Selector2/1, Selector4/1
  Selector3/1 -> Vector Concatenate1/2  "uct y"
  Selector5/1 -> Vector Concatenate2/2  "uct h"
  Uct/1 -> Selector1/1, Selector3/1, Selector5/1
  Selector1/1 -> Vector Concatenate/2  "uct x"
  Vector Concatenate1/1 -> Scope/2
  Vector Concatenate2/1 -> Scope/3
  Selector2/1 -> Vector Concatenate1/1  "mdl y"
  Selector/1 -> Vector Concatenate/1  "mdl x"
  Selector4/1 -> Vector Concatenate2/1  "mdl h"
  Vector Concatenate/1 -> Scope/1

== system MSV_ablf/MSV_w//uncertainty_ABLF/Cmatrix ==
  x2 : Inport
  Add : Sum
  Constant : Constant  Value=0
  Gain : Gain  Gain=-24.6612
  Gain1 : Gain  Gain=25.8
  Gain2 : Gain  Gain=-25.8
  Gain3 : Gain  Gain=24.6612
  Gain4 : Gain  Gain=1.0948
  Matrix Concatenate3 : Concatenate  NumInputs=3  Mode=Multidimensional array
  Matrix Multiply : Product  Multiplication=Matrix(*)
  ROW 2 : Concatenate  NumInputs=3  Mode=Multidimensional array  ConcatenateDimension=2
  ROW1 : Concatenate  NumInputs=3  Mode=Multidimensional array  ConcatenateDimension=2
  ROW3 : Concatenate  NumInputs=3  Mode=Multidimensional array  ConcatenateDimension=2
  Row1[x2] : dspmtrx3/Submatrix  RowSpan=One row  RowStartMode=First  RowStartIndex=1  RowEndMode=Last  RowEndIndex=1  ColSpan=One column  ColStartMode=First  ColStartIndex=1  ColEndMode=Last  ColEndIndex=1
  Row2[x2] : dspmtrx3/Submatrix  RowSpan=One row  RowStartMode=Middle  RowStartIndex=1  RowEndMode=Last  RowEndIndex=1  ColSpan=One column  ColStartMode=First  ColStartIndex=1  ColEndMode=Last  ColEndIndex=1
  Row3[x2] : dspmtrx3/Submatrix  RowSpan=One row  RowStartMode=Last  RowStartIndex=1  RowEndMode=Last  RowEndIndex=1  ColSpan=One column  ColStartMode=First  ColStartIndex=1  ColEndMode=Last  ColEndIndex=1
  C(x2)x2 : Outport
  wires:
  Matrix Multiply/1 -> C(x2)x2/1
  x2/1 -> Row2[x2]/1, Row1[x2]/1, Row3[x2]/1, Matrix Multiply/2  "x2"
  Row3[x2]/1 -> Gain4/1  "ang_vel"
  Add/1 -> ROW3/1
  Gain4/1 -> Add/2
  Row2[x2]/1 -> Gain/1, Gain3/1  "y_vel"
  Gain3/1 -> Add/1
  Gain2/1 -> ROW3/2
  Gain1/1 -> ROW 2/3
  Gain/1 -> ROW1/3
  Matrix Concatenate3/1 -> Matrix Multiply/1  "C(x2)"
  Row1[x2]/1 -> Gain1/1, Gain2/1  "x_vel"
  Constant/1 -> ROW1/1, ROW1/2, ROW 2/1, ROW 2/2, ROW3/3
  ROW3/1 -> Matrix Concatenate3/3
  ROW 2/1 -> Matrix Concatenate3/2
  ROW1/1 -> Matrix Concatenate3/1

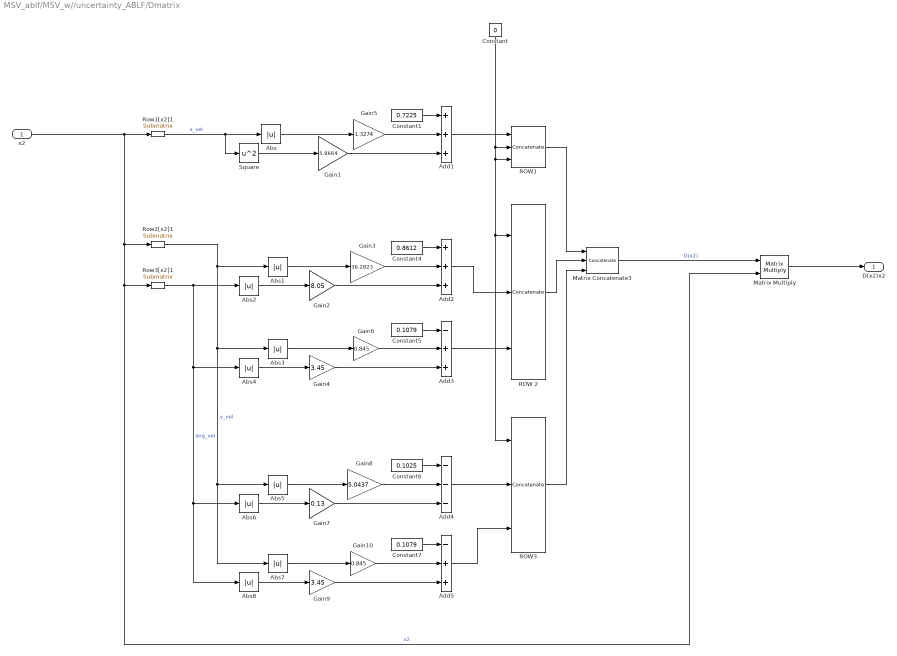
== system MSV_ablf/MSV_w//uncertainty_ABLF/Dmatrix ==
  x2 : Inport
  Abs{,1..8} (9 alike) : Abs
  Add1 : Sum  Inputs=+++
  Add2 : Sum  Inputs=+++
  Add3 : Sum  Inputs=-++
  Add4 : Sum  Inputs=---
  Add5 : Sum  Inputs=-++
  Constant : Constant  Value=0
  Constant1 : Constant  Value=0.7225
  Constant4 : Constant  Value=0.8612
  Constant5 : Constant  Value=0.1079
  Constant6 : Constant  Value=0.1025
  Constant7 : Constant  Value=0.1079
  Gain1 : Gain  Gain=5.8664
  Gain10 : Gain  Gain=0.845
  Gain2 : Gain  Gain=8.05
  Gain3 : Gain  Gain=36.2823
  Gain4 : Gain  Gain=3.45
  Gain5 : Gain  Gain=1.3274
  Gain6 : Gain  Gain=0.845
  Gain7 : Gain  Gain=0.13
  Gain8 : Gain  Gain=5.0437
  Gain9 : Gain  Gain=3.45
  Matrix Concatenate3 : Concatenate  NumInputs=3  Mode=Multidimensional array
  Matrix Multiply : Product  Multiplication=Matrix(*)
  ROW 2 : Concatenate  NumInputs=3  Mode=Multidimensional array  ConcatenateDimension=2
  ROW1 : Concatenate  NumInputs=3  Mode=Multidimensional array  ConcatenateDimension=2
  ROW3 : Concatenate  NumInputs=3  Mode=Multidimensional array  ConcatenateDimension=2
  Row1[x2]1 : dspmtrx3/Submatrix  RowSpan=One row  RowStartMode=First  RowStartIndex=1  RowEndMode=Last  RowEndIndex=1  ColSpan=One column  ColStartMode=First  ColStartIndex=1  ColEndMode=Last  ColEndIndex=1
  Row2[x2]1 : dspmtrx3/Submatrix  RowSpan=One row  RowStartMode=Middle  RowStartIndex=1  RowEndMode=Last  RowEndIndex=1  ColSpan=One column  ColStartMode=First  ColStartIndex=1  ColEndMode=Last  ColEndIndex=1
  Row3[x2]1 : dspmtrx3/Submatrix  RowSpan=One row  RowStartMode=Last  RowStartIndex=1  RowEndMode=Last  RowEndIndex=1  ColSpan=One column  ColStartMode=First  ColStartIndex=1  ColEndMode=Last  ColEndIndex=1
  Square : Math  Operator=square  SaturateOnIntegerOverflow=on
  D(x2)x2 : Outport
  wires:
  Matrix Multiply/1 -> D(x2)x2/1
  x2/1 -> Row1[x2]1/1, Row2[x2]1/1, Row3[x2]1/1, Matrix Multiply/2  "x2"
  Add5/1 -> ROW3/3
  Add4/1 -> ROW3/2
  Abs5/1 -> Gain8/1
  Gain7/1 -> Add4/3
  Gain8/1 -> Add4/2
  Constant6/1 -> Add4/1
  Abs6/1 -> Gain7/1
  Row2[x2]1/1 -> Abs1/1, Abs3/1, Abs5/1, Abs7/1  "y_vel"
  Abs8/1 -> Gain9/1
  Constant7/1 -> Add5/1
  Gain10/1 -> Add5/2
  Gain9/1 -> Add5/3
  Abs7/1 -> Gain10/1
  Row3[x2]1/1 -> Abs2/1, Abs4/1, Abs6/1, Abs8/1  "ang_vel"
  Add3/1 -> ROW 2/3
  Abs3/1 -> Gain6/1
  Gain4/1 -> Add3/3
  Gain6/1 -> Add3/2
  Constant5/1 -> Add3/1
  Abs4/1 -> Gain4/1
  Abs2/1 -> Gain2/1
  Add2/1 -> ROW 2/2
  Constant4/1 -> Add2/1
  Gain3/1 -> Add2/2
  Gain2/1 -> Add2/3
  Abs1/1 -> Gain3/1
  Matrix Concatenate3/1 -> Matrix Multiply/1  "D(x2)"
  Add1/1 -> ROW1/1
  Row1[x2]1/1 -> Square/1, Abs/1  "x_vel"
  Square/1 -> Gain1/1
  Abs/1 -> Gain5/1
  Gain1/1 -> Add1/3
  Gain5/1 -> Add1/2
  Constant1/1 -> Add1/1
  ROW1/1 -> Matrix Concatenate3/1
  ROW 2/1 -> Matrix Concatenate3/2
  ROW3/1 -> Matrix Concatenate3/3
  Constant/1 -> ROW1/2, ROW1/3, ROW3/1, ROW 2/1

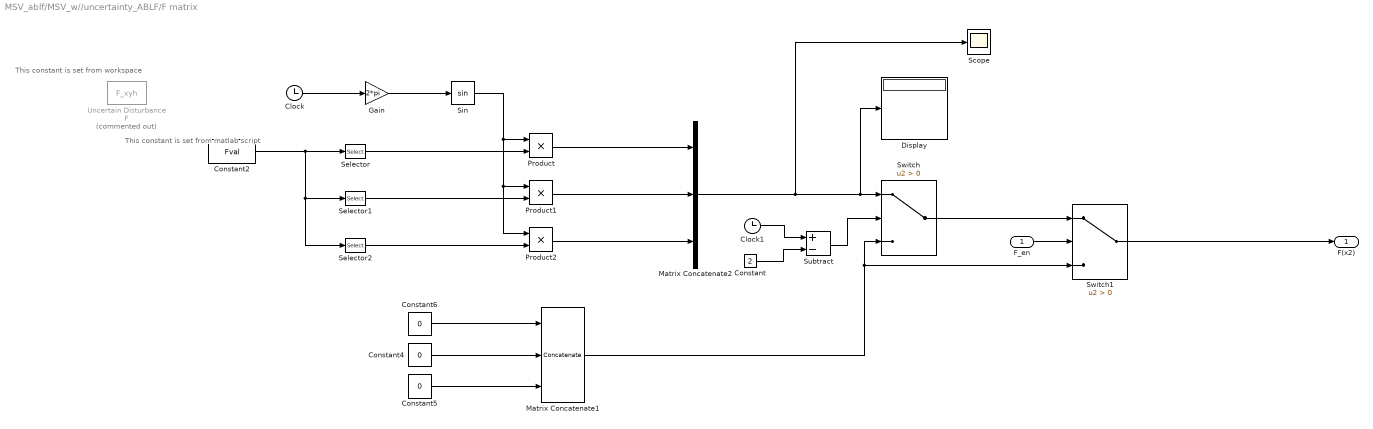
== system MSV_ablf/MSV_w//uncertainty_ABLF/F matrix ==
  note: This constant is set from matlab script
  note: This constant is set from workspace
  F_en : Inport
  Clock : Clock
  Clock1 : Clock
  Constant : Constant  Value=2
  Constant2 : Constant  Value=Fval
  Constant4 : Constant  Value=0
  Constant5 : Constant  Value=0
  Constant6 : Constant  Value=0
  Display : Display
  Gain : Gain  Gain=2*pi
  Matrix Concatenate1 : Concatenate  NumInputs=3  Mode=Multidimensional array
  Matrix Concatenate2 : Concatenate  NumInputs=3  Mode=Multidimensional array
  Product : Product
  Product1 : Product
  Product2 : Product
  Scope : Scope
  Selector : Selector  InputPortWidth=3  IndexOptions=Index vector (dialog)  Indices=1  OutputSizes=1
  Selector1 : Selector  InputPortWidth=3  IndexOptions=Index vector (dialog)  Indices=2  OutputSizes=1
  Selector2 : Selector  InputPortWidth=3  IndexOptions=Index vector (dialog)  Indices=3  OutputSizes=1
  Sin : Trigonometry
  Subtract : Sum  Inputs=+-
  Switch : Switch  Criteria=u2 > Threshold
  Switch1 : Switch  Criteria=u2 > Threshold
  Uncertain Disturbance F : Constant  Commented=on  Value=F_xyh
  F(x2) : Outport
  wires:
  F_en/1 -> Switch1/2
  Switch1/1 -> F(x2)/1
  Constant5/1 -> Matrix Concatenate1/3
  Constant4/1 -> Matrix Concatenate1/2
  Constant6/1 -> Matrix Concatenate1/1
  Matrix Concatenate1/1 -> Switch1/3, Switch/3
  Matrix Concatenate2/1 -> Scope/1, Display/1, Switch/1
  Clock1/1 -> Subtract/1
  Constant/1 -> Subtract/2
  Subtract/1 -> Switch/2
  Switch/1 -> Switch1/1
  Product/1 -> Matrix Concatenate2/1
  Product2/1 -> Matrix Concatenate2/3
  Product1/1 -> Matrix Concatenate2/2
  Sin/1 -> Product1/1, Product2/1, Product/1
  Selector/1 -> Product/2
  Selector1/1 -> Product1/2
  Selector2/1 -> Product2/2
  Gain/1 -> Sin/1
  Clock/1 -> Gain/1
  Constant2/1 -> Selector2/1, Selector1/1, Selector/1

== system MSV_ablf/MSV_w//uncertainty_ABLF/Gmatrix ==
  note: Set to 0 for G(x1) = [ 0 0 0]
  en : Inport
  x13 : Inport  Port=2
  Add g2 : Sum
  Cos : Trigonometry  Operator=cos
  Cos1 : Trigonometry  Operator=cos
  Gain : Gain  Gain=0.2
  Gain1 : Gain  Gain=0.36
  Gain2 : Gain  Gain=0.2
  Gain3 : Gain  Gain=0.36
  Matrix Concatenate : Concatenate  NumInputs=3  Mode=Multidimensional array
  Sin : Trigonometry
  Sin1 : Trigonometry
  Subtract g1 : Sum  Inputs=+-
  Switch : Switch  Criteria=u2 > Threshold
  g1 : Constant  Value=[0 0 0]'  VectorParams1D=off
  g3 : Constant  Value=0.18
  G(x1) : Outport
  wires:
  en/1 -> Switch/2
  g1/1 -> Switch/3
  Matrix Concatenate/1 -> Switch/1
  Switch/1 -> G(x1)/1
  Cos1/1 -> Gain3/1
  Gain3/1 -> Add g2/2
  Sin/1 -> Gain1/1
  g3/1 -> Matrix Concatenate/3
  Gain/1 -> Subtract g1/1
  Cos/1 -> Gain/1
  Subtract g1/1 -> Matrix Concatenate/1
  x13/1 -> Cos/1, Sin/1, Sin1/1, Cos1/1
  Sin1/1 -> Gain2/1
  Add g2/1 -> Matrix Concatenate/2
  Gain1/1 -> Subtract g1/2
  Gain2/1 -> Add g2/1

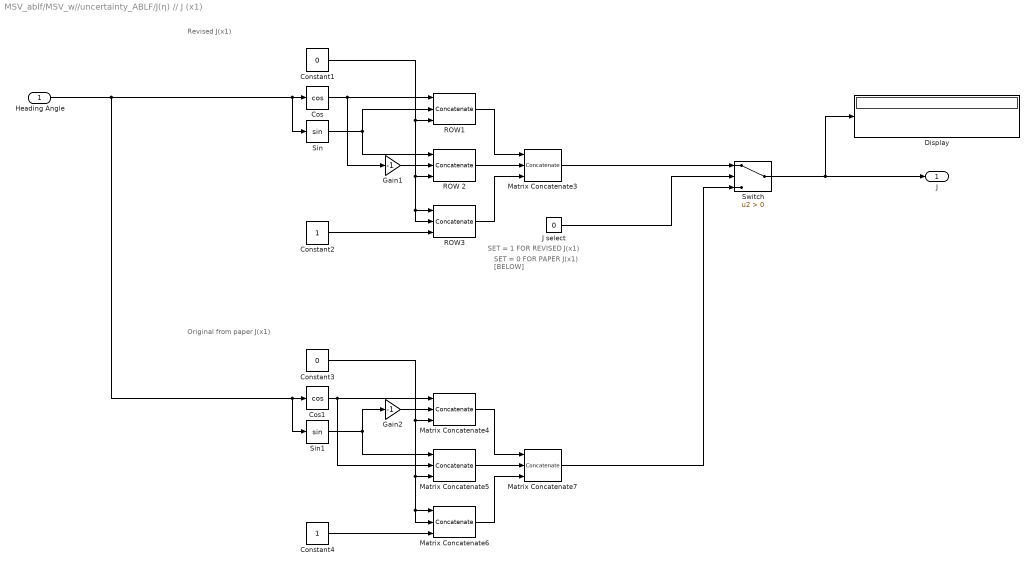
== system MSV_ablf/MSV_w//uncertainty_ABLF/J(η) // J (x1) ==
  note: SET = 0 FOR PAPER J(x1) [BELOW]
  note: Original from paper J(x1)
  note: Revised J(x1)
  note: SET = 1 FOR REVISED J(x1)
  Heading Angle : Inport
  Constant1 : Constant  Value=0
  Constant2 : Constant
  Constant3 : Constant  Value=0
  Constant4 : Constant
  Cos : Trigonometry  Operator=cos  OutputSignalType=real
  Cos1 : Trigonometry  Operator=cos  OutputSignalType=real
  Display : Display
  Gain1 : Gain  Gain=-1
  Gain2 : Gain  Gain=-1
  J select : Constant  Value=0
  Matrix Concatenate3 : Concatenate  NumInputs=3  Mode=Multidimensional array
  Matrix Concatenate4 : Concatenate  NumInputs=3  Mode=Multidimensional array  ConcatenateDimension=2
  Matrix Concatenate5 : Concatenate  NumInputs=3  Mode=Multidimensional array  ConcatenateDimension=2
  Matrix Concatenate6 : Concatenate  NumInputs=3  Mode=Multidimensional array  ConcatenateDimension=2
  Matrix Concatenate7 : Concatenate  NumInputs=3  Mode=Multidimensional array
  ROW 2 : Concatenate  NumInputs=3  Mode=Multidimensional array  ConcatenateDimension=2
  ROW1 : Concatenate  NumInputs=3  Mode=Multidimensional array  ConcatenateDimension=2
  ROW3 : Concatenate  NumInputs=3  Mode=Multidimensional array  ConcatenateDimension=2
  Sin : Trigonometry
  Sin1 : Trigonometry
  Switch : Switch  Criteria=u2 > Threshold
  J : Outport
  wires:
  Gain2/1 -> Matrix Concatenate4/2
  J select/1 -> Switch/2
  Matrix Concatenate7/1 -> Switch/3
  Switch/1 -> J/1, Display/1
  Sin1/1 -> Gain2/1, Matrix Concatenate5/1
  Matrix Concatenate4/1 -> Matrix Concatenate7/1
  Matrix Concatenate5/1 -> Matrix Concatenate7/2
  Constant4/1 -> Matrix Concatenate6/3
  Constant3/1 -> Matrix Concatenate5/3, Matrix Concatenate6/2, Matrix Concatenate6/1, Matrix Concatenate4/3
  Heading Angle/1 -> Cos/1, Sin/1, Sin1/1, Cos1/1
  Matrix Concatenate6/1 -> Matrix Concatenate7/3
  Cos1/1 -> Matrix Concatenate5/2, Matrix Concatenate4/1
  Gain1/1 -> ROW 2/2
  Sin/1 -> ROW 2/1, ROW1/2
  Cos/1 -> Gain1/1, ROW1/1
  Matrix Concatenate3/1 -> Switch/1
  ROW3/1 -> Matrix Concatenate3/3
  Constant1/1 -> ROW1/3, ROW3/1, ROW3/2, ROW 2/3
  Constant2/1 -> ROW3/3
  ROW 2/1 -> Matrix Concatenate3/2
  ROW1/1 -> Matrix Concatenate3/1

== system MSV_ablf/MSV_w//uncertainty_BS/Added Uncertainty ==
  Mdl : Inport
  Uct : Inport  Port=2
  Scope : Scope  NumInputPorts=3
  Selector : Selector  InputPortWidth=3  IndexOptions=Index vector (dialog)  Indices=1  OutputSizes=1
  Selector1 : Selector  InputPortWidth=3  IndexOptions=Index vector (dialog)  Indices=1  OutputSizes=1
  Selector2 : Selector  InputPortWidth=3  IndexOptions=Index vector (dialog)  Indices=2  OutputSizes=1
  Selector3 : Selector  InputPortWidth=3  IndexOptions=Index vector (dialog)  Indices=2  OutputSizes=1
  Selector4 : Selector  InputPortWidth=3  IndexOptions=Index vector (dialog)  Indices=3  OutputSizes=1
  Selector5 : Selector  InputPortWidth=3  IndexOptions=Index vector (dialog)  Indices=3  OutputSizes=1
  Vector Concatenate : Concatenate
  Vector Concatenate1 : Concatenate
  Vector Concatenate2 : Concatenate
  wires:
  Vector Concatenate/1 -> Scope/1
  Selector4/1 -> Vector Concatenate2/1  "mdl h"
  Selector/1 -> Vector Concatenate/1  "mdl x"
  Selector2/1 -> Vector Concatenate1/1  "mdl y"
  Vector Concatenate2/1 -> Scope/3
  Vector Concatenate1/1 -> Scope/2
  Selector1/1 -> Vector Concatenate/2  "uct x"
  Uct/1 -> Selector5/1, Selector3/1, Selector1/1
  Selector5/1 -> Vector Concatenate2/2  "uct h"
  Selector3/1 -> Vector Concatenate1/2  "uct y"
  Mdl/1 -> Selector4/1, Selector2/1, Selector/1

== system MSV_ablf/MSV_w//uncertainty_BS/Cmatrix ==
  x2 : Inport
  Add : Sum
  Constant : Constant  Value=0
  Gain : Gain  Gain=-24.6612
  Gain1 : Gain  Gain=25.8
  Gain2 : Gain  Gain=-25.8
  Gain3 : Gain  Gain=24.6612
  Gain4 : Gain  Gain=1.0948
  Matrix Concatenate3 : Concatenate  NumInputs=3  Mode=Multidimensional array
  Matrix Multiply : Product  Multiplication=Matrix(*)
  ROW 2 : Concatenate  NumInputs=3  Mode=Multidimensional array  ConcatenateDimension=2
  ROW1 : Concatenate  NumInputs=3  Mode=Multidimensional array  ConcatenateDimension=2
  ROW3 : Concatenate  NumInputs=3  Mode=Multidimensional array  ConcatenateDimension=2
  Row1[x2] : dspmtrx3/Submatrix  RowSpan=One row  RowStartMode=First  RowStartIndex=1  RowEndMode=Last  RowEndIndex=1  ColSpan=One column  ColStartMode=First  ColStartIndex=1  ColEndMode=Last  ColEndIndex=1
  Row2[x2] : dspmtrx3/Submatrix  RowSpan=One row  RowStartMode=Middle  RowStartIndex=1  RowEndMode=Last  RowEndIndex=1  ColSpan=One column  ColStartMode=First  ColStartIndex=1  ColEndMode=Last  ColEndIndex=1
  Row3[x2] : dspmtrx3/Submatrix  RowSpan=One row  RowStartMode=Last  RowStartIndex=1  RowEndMode=Last  RowEndIndex=1  ColSpan=One column  ColStartMode=First  ColStartIndex=1  ColEndMode=Last  ColEndIndex=1
  C(x2)x2 : Outport
  wires:
  ROW1/1 -> Matrix Concatenate3/1
  ROW 2/1 -> Matrix Concatenate3/2
  ROW3/1 -> Matrix Concatenate3/3
  Constant/1 -> ROW3/3, ROW 2/2, ROW 2/1, ROW1/2, ROW1/1
  Row1[x2]/1 -> Gain2/1, Gain1/1  "x_vel"
  Matrix Concatenate3/1 -> Matrix Multiply/1  "C(x2)"
  Gain/1 -> ROW1/3
  Gain1/1 -> ROW 2/3
  Gain2/1 -> ROW3/2
  Gain3/1 -> Add/1
  Row2[x2]/1 -> Gain3/1, Gain/1  "y_vel"
  Gain4/1 -> Add/2
  Add/1 -> ROW3/1
  Row3[x2]/1 -> Gain4/1  "ang_vel"
  x2/1 -> Matrix Multiply/2, Row3[x2]/1, Row1[x2]/1, Row2[x2]/1  "x2"
  Matrix Multiply/1 -> C(x2)x2/1

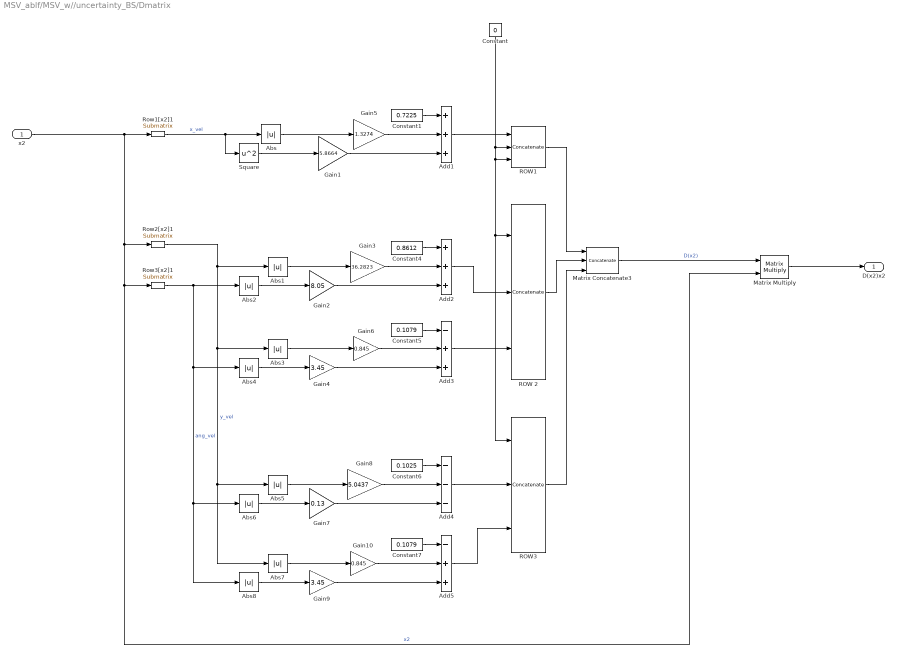
== system MSV_ablf/MSV_w//uncertainty_BS/Dmatrix ==
  x2 : Inport
  Abs{,1..8} (9 alike) : Abs
  Add1 : Sum  Inputs=+++
  Add2 : Sum  Inputs=+++
  Add3 : Sum  Inputs=-++
  Add4 : Sum  Inputs=---
  Add5 : Sum  Inputs=-++
  Constant : Constant  Value=0
  Constant1 : Constant  Value=0.7225
  Constant4 : Constant  Value=0.8612
  Constant5 : Constant  Value=0.1079
  Constant6 : Constant  Value=0.1025
  Constant7 : Constant  Value=0.1079
  Gain1 : Gain  Gain=5.8664
  Gain10 : Gain  Gain=0.845
  Gain2 : Gain  Gain=8.05
  Gain3 : Gain  Gain=36.2823
  Gain4 : Gain  Gain=3.45
  Gain5 : Gain  Gain=1.3274
  Gain6 : Gain  Gain=0.845
  Gain7 : Gain  Gain=0.13
  Gain8 : Gain  Gain=5.0437
  Gain9 : Gain  Gain=3.45
  Matrix Concatenate3 : Concatenate  NumInputs=3  Mode=Multidimensional array
  Matrix Multiply : Product  Multiplication=Matrix(*)
  ROW 2 : Concatenate  NumInputs=3  Mode=Multidimensional array  ConcatenateDimension=2
  ROW1 : Concatenate  NumInputs=3  Mode=Multidimensional array  ConcatenateDimension=2
  ROW3 : Concatenate  NumInputs=3  Mode=Multidimensional array  ConcatenateDimension=2
  Row1[x2]1 : dspmtrx3/Submatrix  RowSpan=One row  RowStartMode=First  RowStartIndex=1  RowEndMode=Last  RowEndIndex=1  ColSpan=One column  ColStartMode=First  ColStartIndex=1  ColEndMode=Last  ColEndIndex=1
  Row2[x2]1 : dspmtrx3/Submatrix  RowSpan=One row  RowStartMode=Middle  RowStartIndex=1  RowEndMode=Last  RowEndIndex=1  ColSpan=One column  ColStartMode=First  ColStartIndex=1  ColEndMode=Last  ColEndIndex=1
  Row3[x2]1 : dspmtrx3/Submatrix  RowSpan=One row  RowStartMode=Last  RowStartIndex=1  RowEndMode=Last  RowEndIndex=1  ColSpan=One column  ColStartMode=First  ColStartIndex=1  ColEndMode=Last  ColEndIndex=1
  Square : Math  Operator=square  SaturateOnIntegerOverflow=on
  D(x2)x2 : Outport
  wires:
  Constant/1 -> ROW 2/1, ROW3/1, ROW1/3, ROW1/2
  ROW3/1 -> Matrix Concatenate3/3
  ROW 2/1 -> Matrix Concatenate3/2
  ROW1/1 -> Matrix Concatenate3/1
  Constant1/1 -> Add1/1
  Gain5/1 -> Add1/2
  Gain1/1 -> Add1/3
  Abs/1 -> Gain5/1
  Square/1 -> Gain1/1
  Row1[x2]1/1 -> Abs/1, Square/1  "x_vel"
  Add1/1 -> ROW1/1
  Matrix Concatenate3/1 -> Matrix Multiply/1  "D(x2)"
  Abs1/1 -> Gain3/1
  Gain2/1 -> Add2/3
  Gain3/1 -> Add2/2
  Constant4/1 -> Add2/1
  Add2/1 -> ROW 2/2
  Abs2/1 -> Gain2/1
  Abs4/1 -> Gain4/1
  Constant5/1 -> Add3/1
  Gain6/1 -> Add3/2
  Gain4/1 -> Add3/3
  Abs3/1 -> Gain6/1
  Add3/1 -> ROW 2/3
  Row3[x2]1/1 -> Abs8/1, Abs6/1, Abs4/1, Abs2/1  "ang_vel"
  Abs7/1 -> Gain10/1
  Gain9/1 -> Add5/3
  Gain10/1 -> Add5/2
  Constant7/1 -> Add5/1
  Abs8/1 -> Gain9/1
  Row2[x2]1/1 -> Abs7/1, Abs5/1, Abs3/1, Abs1/1  "y_vel"
  Abs6/1 -> Gain7/1
  Constant6/1 -> Add4/1
  Gain8/1 -> Add4/2
  Gain7/1 -> Add4/3
  Abs5/1 -> Gain8/1
  Add4/1 -> ROW3/2
  Add5/1 -> ROW3/3
  x2/1 -> Matrix Multiply/2, Row3[x2]1/1, Row2[x2]1/1, Row1[x2]1/1  "x2"
  Matrix Multiply/1 -> D(x2)x2/1

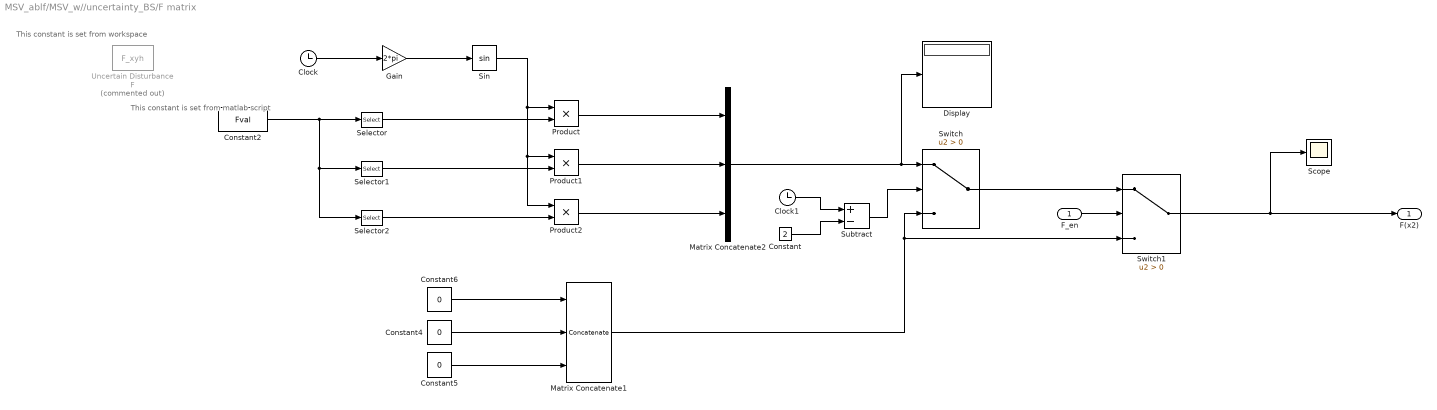
== system MSV_ablf/MSV_w//uncertainty_BS/F matrix ==
  note: This constant is set from matlab script
  note: This constant is set from workspace
  F_en : Inport
  Clock : Clock
  Clock1 : Clock
  Constant : Constant  Value=2
  Constant2 : Constant  Value=Fval
  Constant4 : Constant  Value=0
  Constant5 : Constant  Value=0
  Constant6 : Constant  Value=0
  Display : Display
  Gain : Gain  Gain=2*pi
  Matrix Concatenate1 : Concatenate  NumInputs=3  Mode=Multidimensional array
  Matrix Concatenate2 : Concatenate  NumInputs=3  Mode=Multidimensional array
  Product : Product
  Product1 : Product
  Product2 : Product
  Scope : Scope
  Selector : Selector  InputPortWidth=3  IndexOptions=Index vector (dialog)  Indices=1  OutputSizes=1
  Selector1 : Selector  InputPortWidth=3  IndexOptions=Index vector (dialog)  Indices=2  OutputSizes=1
  Selector2 : Selector  InputPortWidth=3  IndexOptions=Index vector (dialog)  Indices=3  OutputSizes=1
  Sin : Trigonometry
  Subtract : Sum  Inputs=+-
  Switch : Switch  Criteria=u2 > Threshold
  Switch1 : Switch  Criteria=u2 > Threshold
  Uncertain Disturbance F : Constant  Commented=on  Value=F_xyh
  F(x2) : Outport
  wires:
  F_en/1 -> Switch1/2
  Switch1/1 -> Scope/1, F(x2)/1
  Constant5/1 -> Matrix Concatenate1/3
  Constant4/1 -> Matrix Concatenate1/2
  Constant6/1 -> Matrix Concatenate1/1
  Matrix Concatenate1/1 -> Switch1/3, Switch/3
  Matrix Concatenate2/1 -> Display/1, Switch/1
  Clock1/1 -> Subtract/1
  Constant/1 -> Subtract/2
  Subtract/1 -> Switch/2
  Switch/1 -> Switch1/1
  Product/1 -> Matrix Concatenate2/1
  Product2/1 -> Matrix Concatenate2/3
  Product1/1 -> Matrix Concatenate2/2
  Sin/1 -> Product1/1, Product2/1, Product/1
  Selector/1 -> Product/2
  Selector1/1 -> Product1/2
  Selector2/1 -> Product2/2
  Gain/1 -> Sin/1
  Clock/1 -> Gain/1
  Constant2/1 -> Selector2/1, Selector1/1, Selector/1

== system MSV_ablf/MSV_w//uncertainty_BS/Gmatrix ==
  note: Set to 0 for G(x1) = [ 0 0 0]
  en : Inport
  x13 : Inport  Port=2
  Add g2 : Sum
  Cos : Trigonometry  Operator=cos
  Cos1 : Trigonometry  Operator=cos
  Gain : Gain  Gain=0.2
  Gain1 : Gain  Gain=0.36
  Gain2 : Gain  Gain=0.2
  Gain3 : Gain  Gain=0.36
  Matrix Concatenate : Concatenate  NumInputs=3  Mode=Multidimensional array
  Sin : Trigonometry
  Sin1 : Trigonometry
  Subtract g1 : Sum  Inputs=+-
  Switch : Switch  Criteria=u2 > Threshold
  g1 : Constant  Value=[0 0 0]'  VectorParams1D=off
  g3 : Constant  Value=0.18
  G(x1) : Outport
  wires:
  Gain2/1 -> Add g2/1
  Gain1/1 -> Subtract g1/2
  Add g2/1 -> Matrix Concatenate/2
  Sin1/1 -> Gain2/1
  x13/1 -> Cos1/1, Sin1/1, Sin/1, Cos/1
  Subtract g1/1 -> Matrix Concatenate/1
  Cos/1 -> Gain/1
  Gain/1 -> Subtract g1/1
  g3/1 -> Matrix Concatenate/3
  Sin/1 -> Gain1/1
  Gain3/1 -> Add g2/2
  Cos1/1 -> Gain3/1
  Switch/1 -> G(x1)/1
  Matrix Concatenate/1 -> Switch/1
  g1/1 -> Switch/3
  en/1 -> Switch/2
